simulink model "subsystem_validation_turb"  (R2020a)
settings: Solver=VariableStepAuto  StartTime=0.0  StopTime=10.0  RelTol=1e-3
values from neighbouring files (symbols this model uses):
  BSR_max = k(2)    [Project2A.m]
  cp_exh = gamma_exh*cv_exh    [Init_Project1.m]    (also in Project2A.m = 1213.3)
  eta_t_max = k(1)    [Project2A.m]
  etaTmin = min(turb.etaT)/2    [Project2A.m]
  gamma_exh = EngineMap.airfuel.gamma_exh    [Init_Project1.m]    (also in Project2A.m = 1.3)
  k_0 = k(1)    [Project2A.m]
  k_1 = k(2)    [Project2A.m]
  Nt = TSP.*sqrt(T03)    [Project2A.m]
  p03 = p04./PiT    [Project2A.m]
  p04 = turb.p04    [Project2A.m]
  rTurb = dTurb/2    (= 0.0261)    [Project2A.m]
  T03 = turb.T03    [Project2A.m]
settings Model: Creator=David Wiman  LastModifiedBy=David Wiman

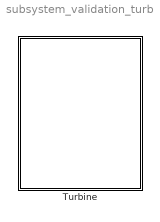
== system subsystem_validation_turb ==
  Turbine : Subsystem

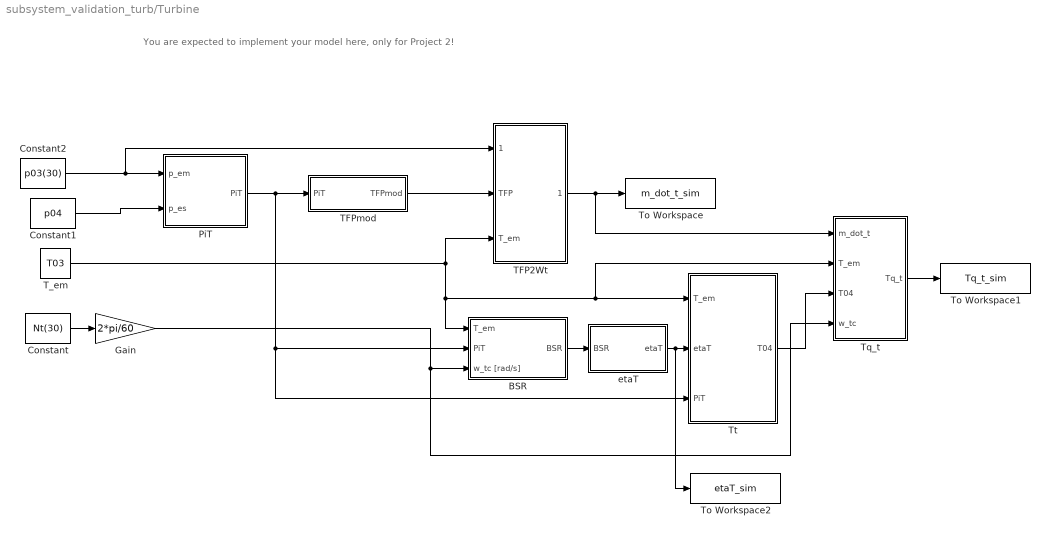
== system subsystem_validation_turb/Turbine ==
  note: You are expected to implement your model here, only for Project 2!
  BSR : Subsystem
  Constant : Constant  Value=Nt(30)
  Constant1 : Constant  Value=p04
  Constant2 : Constant  Value=p03(30)
  Gain : Gain  Gain=2*pi/60
  PiT : Subsystem
  TFP2Wt : Subsystem
  TFPmod : Subsystem
  T_em : Constant  Value=T03
  To Workspace : ToWorkspace  VariableName=m_dot_t_sim  SampleTime=-1
  To Workspace1 : ToWorkspace  VariableName=Tq_t_sim  SampleTime=-1
  To Workspace2 : ToWorkspace  VariableName=etaT_sim  SampleTime=-1
  Tq_t : Subsystem
  Tt : Subsystem
  etaT : Subsystem
  wires:
  BSR/1(BSR) -> etaT/1(BSR)
  Constant2/1 -> PiT/1(p_em), TFP2Wt/1(p_em [Pa])
  Gain/1 -> BSR/3(w_tc [rad/s]), Tq_t/4(w_tc)
  T_em/1 -> TFP2Wt/3(T_em), BSR/1(T_em), Tq_t/2(T_em), Tt/1(T_em)
  TFPmod/1(TFPmod) -> TFP2Wt/2(TFP)
  TFP2Wt/1(m_dot_t) -> To Workspace/1, Tq_t/1(m_dot_t)
  etaT/1(etaT) -> To Workspace2/1, Tt/2(etaT)
  Tq_t/1(Tq_t) -> To Workspace1/1
  Tt/1(T04) -> Tq_t/3(T04)
  PiT/1(PiT) -> TFPmod/1(PiT), BSR/2(PiT), Tt/3(PiT)
  Constant/1 -> Gain/1
  Constant1/1 -> PiT/2(p_es)

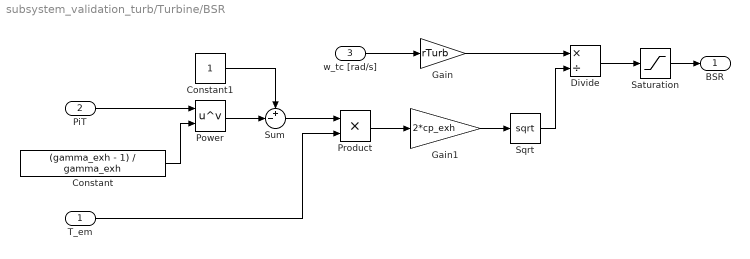
== system subsystem_validation_turb/Turbine/BSR ==
  T_em : Inport
  PiT : Inport  Port=2
  w_tc [rad/s] : Inport  Port=3
  Constant : Constant  Value=(gamma_exh - 1) / gamma_exh
  Constant1 : Constant
  Divide : Product  Inputs=*/
  Gain : Gain  Gain=rTurb
  Gain1 : Gain  Gain=2*cp_exh
  Power : Math  Operator=pow  SaturateOnIntegerOverflow=on
  Product : Product
  Saturation : Saturate  UpperLimit=1  LowerLimit=0.1
  Sqrt : Sqrt  SaturateOnIntegerOverflow=on
  Sum : Sum  Inputs=+-|
  BSR : Outport
  wires:
  w_tc [rad/s]/1 -> Gain/1
  PiT/1 -> Power/1
  T_em/1 -> Product/2
  Divide/1 -> Saturation/1
  Saturation/1 -> BSR/1
  Constant/1 -> Power/2
  Power/1 -> Sum/2
  Constant1/1 -> Sum/1
  Sum/1 -> Product/1
  Product/1 -> Gain1/1
  Gain1/1 -> Sqrt/1
  Sqrt/1 -> Divide/2
  Gain/1 -> Divide/1

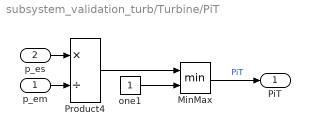
== system subsystem_validation_turb/Turbine/PiT ==
  p_em : Inport
  p_es : Inport  Port=2
  MinMax : MinMax  Inputs=2
  Product4 : Product  Inputs=*/  RndMeth=Zero
  one1 : Constant
  PiT : Outport
  wires:
  Product4/1 -> MinMax/1
  one1/1 -> MinMax/2
  p_em/1 -> Product4/2
  MinMax/1 -> PiT/1  "PiT"
  p_es/1 -> Product4/1

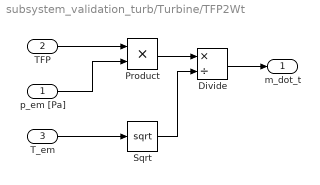
== system subsystem_validation_turb/Turbine/TFP2Wt ==
  p_em [Pa] : Inport
  TFP : Inport  Port=2
  T_em : Inport  Port=3
  Divide : Product  Inputs=*/
  Product : Product
  Sqrt : Sqrt  SaturateOnIntegerOverflow=on
  m_dot_t : Outport
  wires:
  p_em [Pa]/1 -> Product/2
  T_em/1 -> Sqrt/1
  TFP/1 -> Product/1
  Divide/1 -> m_dot_t/1
  Product/1 -> Divide/1
  Sqrt/1 -> Divide/2

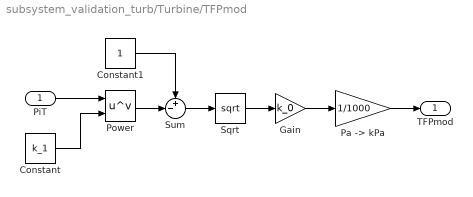
== system subsystem_validation_turb/Turbine/TFPmod ==
  PiT : Inport
  Constant : Constant  Value=k_1
  Constant1 : Constant
  Gain : Gain  Gain=k_0
  "Pa -> kPa" : Gain  Gain=1/1000
  Power : Math  Operator=pow  SaturateOnIntegerOverflow=on
  Sqrt : Sqrt  SaturateOnIntegerOverflow=on
  Sum : Sum  Inputs=+-|
  TFPmod : Outport
  wires:
  PiT/1 -> Power/1
  Constant/1 -> Power/2
  Power/1 -> Sum/2
  Constant1/1 -> Sum/1
  Sum/1 -> Sqrt/1
  Sqrt/1 -> Gain/1
  Gain/1 -> "Pa -> kPa"/1
  "Pa -> kPa"/1 -> TFPmod/1

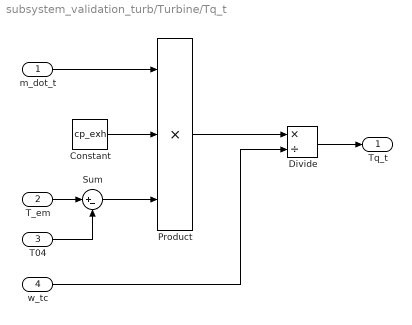
== system subsystem_validation_turb/Turbine/Tq_t ==
  m_dot_t : Inport
  T_em : Inport  Port=2
  T04 : Inport  Port=3
  w_tc : Inport  Port=4
  Constant : Constant  Value=cp_exh
  Divide : Product  Inputs=*/
  Product : Product  Inputs=3
  Sum : Sum  Inputs=|+-
  Tq_t : Outport
  wires:
  Divide/1 -> Tq_t/1
  Constant/1 -> Product/2
  Product/1 -> Divide/1
  Sum/1 -> Product/3
  w_tc/1 -> Divide/2
  m_dot_t/1 -> Product/1
  T_em/1 -> Sum/1
  T04/1 -> Sum/2

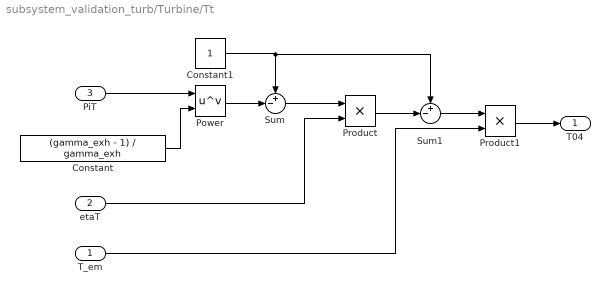
== system subsystem_validation_turb/Turbine/Tt ==
  T_em : Inport
  etaT : Inport  Port=2
  PiT : Inport  Port=3
  Constant : Constant  Value=(gamma_exh - 1) / gamma_exh
  Constant1 : Constant
  Power : Math  Operator=pow  SaturateOnIntegerOverflow=on
  Product : Product
  Product1 : Product
  Sum : Sum  Inputs=+-|
  Sum1 : Sum  Inputs=+-|
  T04 : Outport
  wires:
  T_em/1 -> Product1/2
  etaT/1 -> Product/2
  Product1/1 -> T04/1
  Power/1 -> Sum/2
  Constant/1 -> Power/2
  Constant1/1 -> Sum1/1, Sum/1
  PiT/1 -> Power/1
  Sum/1 -> Product/1
  Product/1 -> Sum1/2
  Sum1/1 -> Product1/1

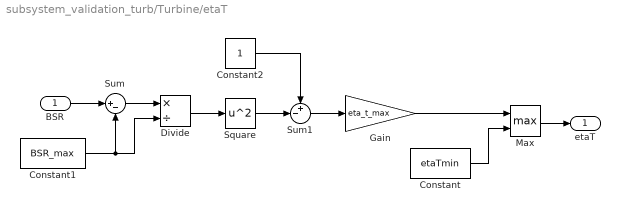
== system subsystem_validation_turb/Turbine/etaT ==
  BSR : Inport
  Constant : Constant  Value=etaTmin
  Constant1 : Constant  Value=BSR_max
  Constant2 : Constant
  Divide : Product  Inputs=*/
  Gain : Gain  Gain=eta_t_max
  Max : MinMax  Function=max  Inputs=2
  Square : Math  Operator=square  SaturateOnIntegerOverflow=on
  Sum : Sum  Inputs=|+-
  Sum1 : Sum  Inputs=+-|
  etaT : Outport
  wires:
  Max/1 -> etaT/1
  Constant/1 -> Max/2
  BSR/1 -> Sum/1
  Gain/1 -> Max/1
  Constant1/1 -> Sum/2, Divide/2
  Sum/1 -> Divide/1
  Divide/1 -> Square/1
  Square/1 -> Sum1/2
  Constant2/1 -> Sum1/1
  Sum1/1 -> Gain/1
